simulink model "Lab3_Start"  (R2017a)
settings: Solver=VariableStepAuto  StartTime=0.0  StopTime=1  RelTol=1e-3
libraries: fl_lib x13, nesl_utility x7, elec_lib x1
settings Model: Creator=Nic  LastModifiedBy=Nic

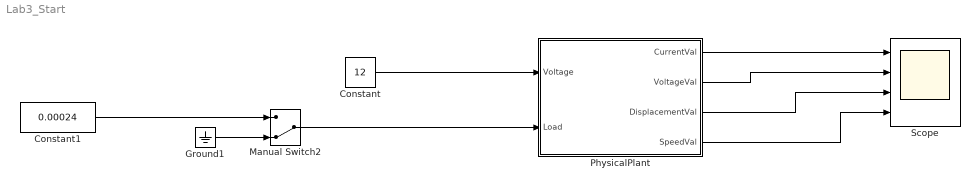
== system Lab3_Start ==
  Constant : Constant  Value=12
  Constant1 : Constant  Value=0.00024
  Ground1 : Ground
  Manual Switch2 : ManualSwitch  CurrentSetting=0
  PhysicalPlant : Subsystem
  Scope : Scope  NumInputPorts=4
  wires:
  PhysicalPlant/1(CurrentVal) -> Scope/1
  PhysicalPlant/2(VoltageVal) -> Scope/2
  PhysicalPlant/3(DisplacementVal) -> Scope/3
  PhysicalPlant/4(SpeedVal) -> Scope/4
  Constant/1 -> PhysicalPlant/1(Voltage)
  Manual Switch2/1 -> PhysicalPlant/2(Load)
  Ground1/1 -> Manual Switch2/2
  Constant1/1 -> Manual Switch2/1

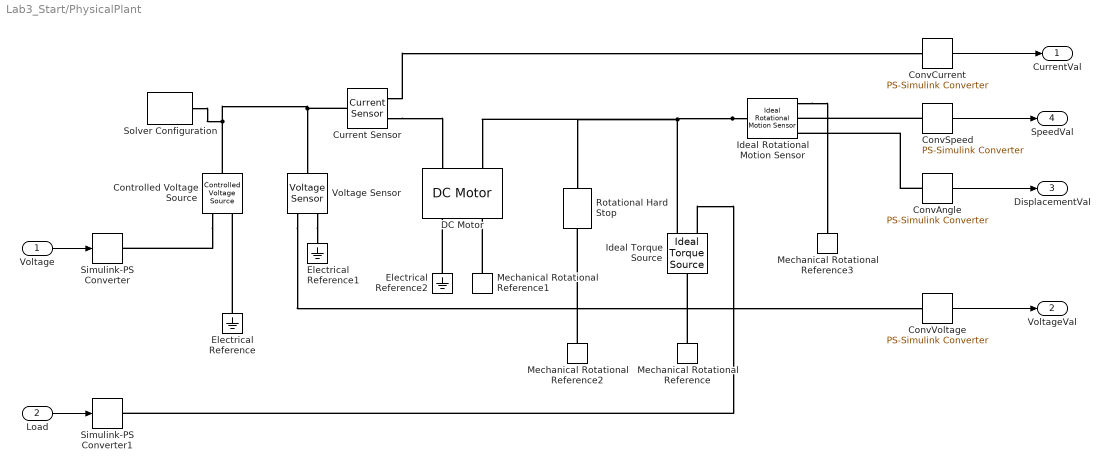
== system Lab3_Start/PhysicalPlant ==
  Voltage : Inport
  Load : Inport  Port=2
  Controlled Voltage Source : fl_lib/Electrical/Electrical Sources/Controlled Voltage Source
  ConvAngle : nesl_utility/PS-Simulink Converter  PhysicalDomain=network_engine_domain  SubClassName=ps_output  LeftPortType=input  RightPortType=output  PseudoPeriodic=off  Frequencies=[]  Unit=rad  AffineConversion=off
  ConvCurrent : nesl_utility/PS-Simulink Converter  PhysicalDomain=network_engine_domain  SubClassName=ps_output  LeftPortType=input  RightPortType=output  PseudoPeriodic=off  Frequencies=[]  Unit=A  AffineConversion=off
  ConvSpeed : nesl_utility/PS-Simulink Converter  PhysicalDomain=network_engine_domain  SubClassName=ps_output  LeftPortType=input  RightPortType=output  PseudoPeriodic=off  Frequencies=[]  Unit=rad/s  AffineConversion=off
  ConvVoltage : nesl_utility/PS-Simulink Converter  PhysicalDomain=network_engine_domain  SubClassName=ps_output  LeftPortType=input  RightPortType=output  PseudoPeriodic=off  Frequencies=[]  Unit=V  AffineConversion=off
  Current Sensor : fl_lib/Electrical/Electrical Sensors/Current Sensor
  DC Motor : elec_lib/Actuators & Drivers/Rotational Actuators/DC Motor  parameterization=1  Ra=0.83 Ohm  La=0.63 mH  emf_or_torque=1  Kv=0.0182 V/(rad/s)  Ki=6.876e-4 N*m/A  T_stall=2.4e-4 N*m  w_max=1.91e+4 rpm  w_rated=1.5e+4 rpm  P_rated=0.08 W  V_rated=1.5 V  J=4.2e-6 kg*m^2  lam_param=1  lam=2.6e-06 N*m/(rad/s)  i_noload=0 A  V_i_noload=1.5 V  speed0=0 rpm  alpha=0.00393 1/K  Tmeas=25 degC  thermal_mass=100 J/K  initial_temperature=25 degC
  Electrical Reference : fl_lib/Electrical/Electrical Elements/Electrical Reference
  Electrical Reference1 : fl_lib/Electrical/Electrical Elements/Electrical Reference
  Electrical Reference2 : fl_lib/Electrical/Electrical Elements/Electrical Reference
  Ideal Rotational Motion Sensor : fl_lib/Mechanical/Mechanical Sensors/Ideal Rotational Motion Sensor  offset=0 rad
  Ideal Torque Source : fl_lib/Mechanical/Mechanical Sources/Ideal Torque Source
  Mechanical Rotational Reference{,1..3} (4 alike) : fl_lib/Mechanical/Rotational Elements/Mechanical Rotational Reference
  Rotational Hard Stop : fl_lib/Mechanical/Rotational Elements/Rotational Hard Stop  upper_bnd=10000 rad  lower_bnd=0 rad  stiff_up=1e3 N*m/rad  stiff_low=1e3 N*m/rad  D_up=0.01 N*m/(rad/s)  D_low=0.01 N*m/(rad/s)  w_specify=off  w_priority=None  w=0 rad/s  w_nominal_specify=off  w_nominal_unit=rad/s  w_nominal_value=1  t_specify=off  t_priority=None  t=0 N*m  t_nominal_specify=off  t_nominal_unit=N*m  t_nominal_value=1  phi_specify=off  phi_priority=None  phi=0 rad  phi_nominal_specify=off  phi_nominal_unit=rad  phi_nominal_value=1
      settings: SourceProductName=Simscape  SourceProductBaseCode=SS
  Simulink-PS Converter : nesl_utility/Simulink-PS Converter  PhysicalDomain=network_engine_domain  SubClassName=ps_input  LeftPortType=input  RightPortType=output  PseudoPeriodic=off  Frequencies=[]  NoiseDistribution=none  NoiseParameters=[]  Unit=V  AffineConversion=off  FilteringAndDerivatives=provide  SimscapeFilterOrder=1  InputFilterTimeConstant=0.001  UdotUserProvided=0
  Simulink-PS Converter1 : nesl_utility/Simulink-PS Converter  PhysicalDomain=network_engine_domain  SubClassName=ps_input  LeftPortType=input  RightPortType=output  PseudoPeriodic=off  Frequencies=[]  NoiseDistribution=none  NoiseParameters=[]  Unit=N*m  AffineConversion=off  FilteringAndDerivatives=provide  SimscapeFilterOrder=1  InputFilterTimeConstant=0.001  UdotUserProvided=0
  Solver Configuration : nesl_utility/Solver Configuration  PhysicalDomain=network_engine_domain  SubClassName=solver  LeftPortType=input  RightPortType=generic  Accelerate=off  Tones=[]  Harmonics=[]  SimulateNoise=off  Profile=off  UseLocalSampling=off  EnableSwitchedLinearOptims=on  FrequencyDomain=off  UseCCode=off  RelTol=0.001  AbsTol=1e-06  MinStep=1e-09  ToWorkspace=off  RevertToSquareIcSolve=off  NumHomotopyIterations=100  PhasorMode=off  PhasorModeNumHarmonics=1  OverrideAbsTol=off  DoDC=off  ResidualTolerance=1e-09  UseLocalSolver=off  LocalSolverChoice=NE_BACKWARD_EULER_ADVANCER  LocalSolverSampleTime=0.001  DoFixedCost=off  MaxNonlinIter=3  MaxModeIter=2  LinearAlgebra=Sparse  DelaysMemoryBudget=1024  AutomaticFiltering=on  FilteringTimeConstant=0.001
  Voltage Sensor : fl_lib/Electrical/Electrical Sensors/Voltage Sensor
  CurrentVal : Outport
  VoltageVal : Outport  Port=2
  DisplacementVal : Outport  Port=3
  SpeedVal : Outport  Port=4
  wires:
  ConvCurrent/1 -> CurrentVal/1
  Load/1 -> Simulink-PS Converter1/1
  Voltage/1 -> Simulink-PS Converter/1
  ConvVoltage/1 -> VoltageVal/1
  ConvSpeed/1 -> SpeedVal/1
  ConvAngle/1 -> DisplacementVal/1
  connections:
  Mechanical Rotational Reference1/LConn1 -- DC Motor/RConn2
  Mechanical Rotational Reference2/LConn1 -- Rotational Hard Stop/RConn1
  Ideal Rotational Motion Sensor/RConn1 -- Mechanical Rotational Reference3/LConn1
  Electrical Reference2/LConn1 -- DC Motor/RConn1
  Controlled Voltage Source/LConn1 -- Solver Configuration/RConn1 -- Current Sensor/LConn1 -- Voltage Sensor/LConn1
  Ideal Rotational Motion Sensor/LConn1 -- Ideal Torque Source/RConn2 -- Rotational Hard Stop/LConn1 -- DC Motor/LConn2
  Controlled Voltage Source/RConn1 -- Simulink-PS Converter/RConn1
  Current Sensor/RConn1 -- ConvCurrent/LConn1
  Voltage Sensor/RConn2 -- Electrical Reference1/LConn1
  Mechanical Rotational Reference/LConn1 -- Ideal Torque Source/LConn1
  Ideal Torque Source/RConn1 -- Simulink-PS Converter1/RConn1
  Current Sensor/RConn2 -- DC Motor/LConn1
  Voltage Sensor/RConn1 -- ConvVoltage/LConn1
  Electrical Reference/LConn1 -- Controlled Voltage Source/RConn2
  ConvSpeed/LConn1 -- Ideal Rotational Motion Sensor/RConn2
  ConvAngle/LConn1 -- Ideal Rotational Motion Sensor/RConn3
